simulink model "ciagly_model_dynamiczny"  (R2021a)
settings: Solver=VariableStepAuto  StartTime=0.0  StopTime=10.0  RelTol=1e-3
values from neighbouring files (symbols this model uses):
  a1 = 0.32    [Wartosci_w_zadaniu.m]    (also in zad_4.m)
  a2 = 0.45    [Wartosci_w_zadaniu.m]    (also in zad_4.m)
  a3 = -0.29    [Wartosci_w_zadaniu.m]    (also in zad_4.m)
  a4 = -0.1    [Wartosci_w_zadaniu.m]    (also in zad_4.m)
  K = 2    [Wartosci_w_zadaniu.m]    (also in zad_4.m)
  T1 = 5    [Wartosci_w_zadaniu.m]    (also in zad_4.m)
  T2 = 8    [Wartosci_w_zadaniu.m]    (also in zad_4.m)
settings Model: Creator=ADMIN  LastModifiedBy=ADMIN

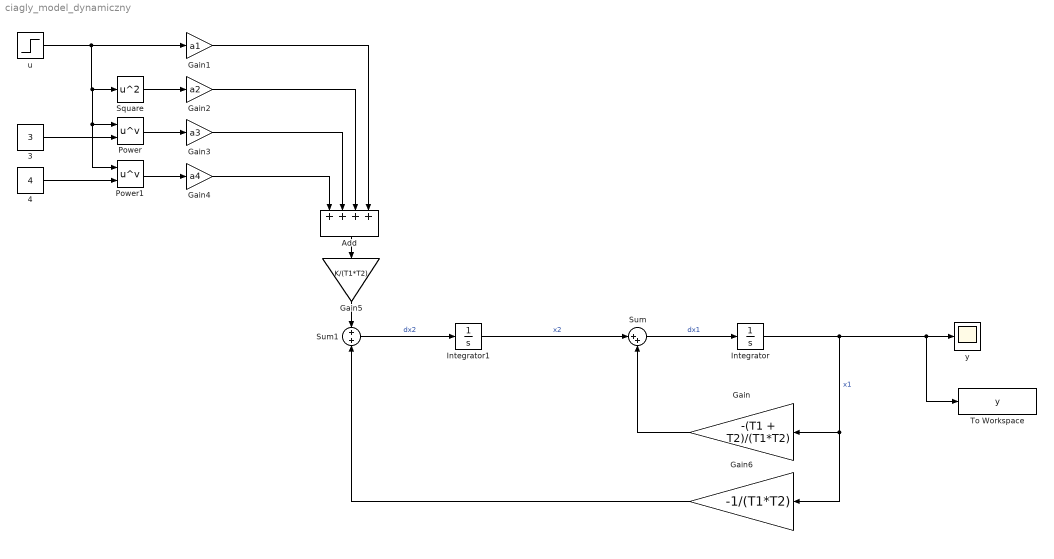
== system ciagly_model_dynamiczny ==
  " 3" : Constant  Value=3
  4 : Constant  Value=4
  Add : Sum  Inputs=++++
  Gain : Gain  Gain=-(T1 + T2)/(T1*T2)
  Gain1 : Gain  Gain=a1
  Gain2 : Gain  Gain=a2
  Gain3 : Gain  Gain=a3
  Gain4 : Gain  Gain=a4
  Gain5 : Gain  Gain=K/(T1*T2)
  Gain6 : Gain  Gain=-1/(T1*T2)
  Integrator : Integrator
  Integrator1 : Integrator
  Power : Math  Operator=pow  SaturateOnIntegerOverflow=on
  Power1 : Math  Operator=pow  SaturateOnIntegerOverflow=on
  Square : Math  Operator=square  SaturateOnIntegerOverflow=on
  Sum : Sum  Inputs=|++
  Sum1 : Sum
  To Workspace : ToWorkspace  VariableName=y  SaveFormat=Timeseries  SampleTime=-1
  u : Step  SampleTime=0
  y : Scope
  wires:
  Gain6/1 -> Sum1/2
  4/1 -> Power1/2
  Power1/1 -> Gain4/1
  u/1 -> Power1/1, Power/1, Square/1, Gain1/1
  Gain4/1 -> Add/1
  Gain1/1 -> Add/4
  " 3"/1 -> Power/2
  Power/1 -> Gain3/1
  Gain2/1 -> Add/3
  Sum/1 -> Integrator/1  "dx1"
  Integrator1/1 -> Sum/1  "x2"
  Sum1/1 -> Integrator1/1  "dx2"
  Gain5/1 -> Sum1/1
  Add/1 -> Gain5/1
  Integrator/1 -> Gain6/1, Gain/1, To Workspace/1, y/1  "x1"
  Gain3/1 -> Add/2
  Square/1 -> Gain2/1
  Gain/1 -> Sum/2
